simulink model "bike_to_point"  (R2022b)
settings: Solver=VariableStepAuto  StartTime=0.0  StopTime=12  RelTol=1e-3
model workspace (MAT data in the model file):
  L = 1
  xo = [10 0 0]
undefined symbols (not defined in the file): magnitude
libraries: simulink x1
settings Model: Creator=cesguti  LastModifiedBy=cesguti

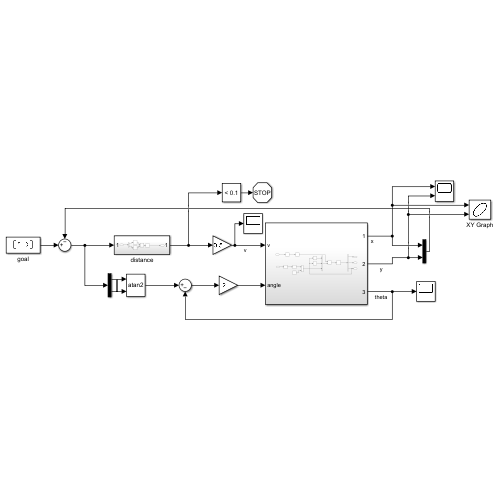
[thumbnail: Simulink's stored preview of the top-level diagram]
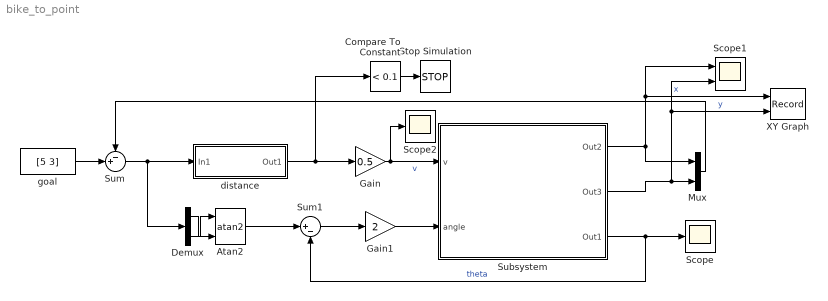
== system bike_to_point ==
  Atan2 : Trigonometry  Operator=atan2
  Compare To Constant : simulink/Logic and Bit Operations/Compare To Constant  relop=<  const=0.1  OutDataTypeStr=boolean
  Demux : Demux  Outputs=2
  Gain : Gain  Gain=0.5
  Gain1 : Gain  Gain=2
  Mux : Mux  Inputs=2
  Scope : Scope
  Scope1 : Scope  NumInputPorts=2
  Scope2 : Scope
  Stop Simulation : Stop
  Subsystem : Subsystem
  Sum : Sum  Inputs=-+|
  Sum1 : Sum  Inputs=|+-
  XY Graph : Record  FileSettingsInternal="{\"entries\":[{\"content\":{\"excelSettings\":{\"content\":{},\"type\":\"Streamout.ExcelSettings\"}},\"type\":\"Streamout.FileSettingStorage\",\"uuid\":\"2cee2774-39ed-4ba8-beb7-37b5c0c4969f\"}],\"packageUris\":[\"http://schema.mathworks.com/mf0/streamout_blocks/R2020a\"],\"version\":\"1.0\"}"  Layout=[1 1]  SignalsInternal="{\"entries\":[{\"content\":{\"signals\":[{\"content\":{\"blockPath\":[\"bike_to_point/XY Graph\"],\"channel\":[],\"dimensions\":[1],\"domain\":\"bike_to_point/XY Graph\",\"lineColor\":\"#a2142f\",\"plots\":[1],\"port\":1,\"sid\":[\"\"],\"signalID\":1385,\"signalName\":\"x\"},\"type\":\"RecordBlkView.Signal\",\"uuid\":\"0fc629dc-b9e7-4b5b-8602-d589ff0061e5\"},{\"content\":{\"blockPath\":[\"bike_to_point/XY Graph\"],\"channel\":[],\"dimensions\":[1],\"domain\":\"bike_to_point/XY Graph\",\"lineColor\":\"#139fff\",\"plots\":[1],\"port\":2,\"sid\":[\"\"],\"signalID\":1389,\"signalName\":\"y\"},\"type\":\"RecordBlkView.Signal\",\"uuid\":\"ae6432e5-62e4-4c00-ab71-a2109088d13c\"}]},\"type\":\"RecordBlkView.InputSignals\",\"uuid\":\"7930c1ef-6bfe-4257-ad38-cffde8761aad\"}],\"packageUris\":[\"http://schema.mathworks.com/mf0/streamout_blocks/R2020a\"],\"version\":\"1.0\"}"  VisualizationBindings="{\"xyplotplugin\":{\"info\":[{\"series\":[{\"bindingParametersList\":[{\"parameter\":\"X-Axis\",\"signalID\":1385,\"signalName\":\"x\"},{\"parameter\":\"Y-Axis\",\"signalID\":1389,\"signalName\":\"y\"}],\"seriesID\":18119}],\"subplotID\":1}]}}"  CompatibilityTag=XY
  distance : Subsystem
  goal : Constant  Value=[5 3]
  wires:
  Gain/1 -> Scope2/1, Subsystem/1(v)  "v"
  Sum/1 -> Demux/1, distance/1(In1)
  distance/1(Out1) -> Compare To Constant/1, Gain/1
  Gain1/1 -> Subsystem/2(angle)
  Sum1/1 -> Gain1/1
  Subsystem/1(Out2) -> XY Graph/1, Scope1/1, Mux/1  "x"
  Subsystem/2(Out3) -> XY Graph/2, Scope1/2, Mux/2  "y"
  Mux/1 -> Sum/1
  goal/1 -> Sum/2
  Atan2/1 -> Sum1/1
  Subsystem/3(Out1) -> Scope/1, Sum1/2  "theta"
  Compare To Constant/1 -> Stop Simulation/1
  Demux/1 -> Atan2/2
  Demux/2 -> Atan2/1

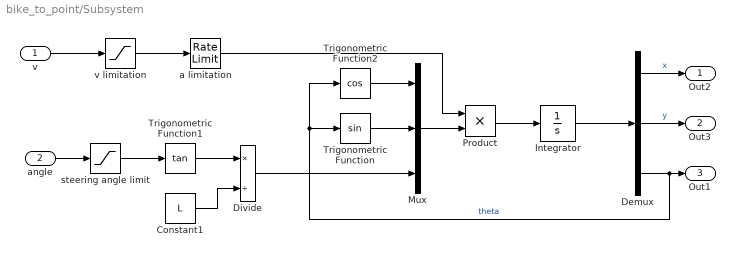
== system bike_to_point/Subsystem ==
  v : Inport
  angle : Inport  Port=2
  Constant1 : Constant  Value=L
  Demux : Demux  Outputs=3
  Divide : Product  Inputs=*/
  Integrator : Integrator  InitialCondition=xo
  Mux : Mux  Inputs=3
  Product : Product
  Trigonometric Function : Trigonometry
  Trigonometric Function1 : Trigonometry  Operator=tan
  Trigonometric Function2 : Trigonometry  Operator=cos
  a limitation : RateLimiter  SampleTimeMode=inherited
  steering angle limit : Saturate  UpperLimit=deg2rad(60)  LowerLimit=deg2rad(-60)
  v limitation : Saturate  UpperLimit=1  LowerLimit=0
  Out2 : Outport
  Out3 : Outport  Port=2
  Out1 : Outport  Port=3
  wires:
  steering angle limit/1 -> Trigonometric Function1/1
  Product/1 -> Integrator/1
  Divide/1 -> Mux/3
  Trigonometric Function/1 -> Mux/2
  v/1 -> v limitation/1
  Constant1/1 -> Divide/2
  Mux/1 -> Product/2
  Trigonometric Function1/1 -> Divide/1
  Trigonometric Function2/1 -> Mux/1
  v limitation/1 -> a limitation/1
  Integrator/1 -> Demux/1
  angle/1 -> steering angle limit/1
  Demux/3 -> Out1/1, Trigonometric Function/1, Trigonometric Function2/1  "theta"
  a limitation/1 -> Product/1
  Demux/1 -> Out2/1  "x"
  Demux/2 -> Out3/1  "y"

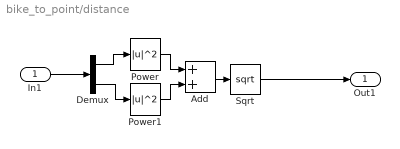
== system bike_to_point/distance ==
  In1 : Inport
  Add : Sum
  Demux : Demux  Outputs=2
  Power : Math  Operator=magnitude^2
  Power1 : Math  Operator=magnitude^2
  Sqrt : Sqrt
  Out1 : Outport
  wires:
  In1/1 -> Demux/1
  Sqrt/1 -> Out1/1
  Demux/1 -> Power/1
  Power1/1 -> Add/2
  Demux/2 -> Power1/1
  Add/1 -> Sqrt/1
  Power/1 -> Add/1
